simulink model "SimulinkAnalysisofCheetahTail"  (R2022a)
settings: Solver=ode4  StartTime=0.0  StopTime=1.5  FixedStep=0.001  RelTol=1e-3
undefined symbols (not defined in the file): B_cg_H, B_con_H, B_con_L, bar_len, cd_table, Cf, cl_table, g, gear_ratio, int_point_bar, int_point_tail, ITail, M_add, M_cg_H, M_cg_L, M_cg_W, Mb, Mm, Mt, psi3, rho, T_cg_H, T_fur_gap, T_length, T_width_major, T_width_minor, th2_initial, torque_constant, uncertainty_Forces, uncertainty_Position, Vf, windspeed
(part 15 of 21)

== matlab function SimulinkAnalysisofCheetahTail/Model/Forces/NonConstraintForceMatrix_tail_4 ==
  data: B_con_H parameter; B_con_L parameter; Cd input; Cl input; Q_tail_4 output; M_cg_H parameter; M_cg_L parameter; M_cg_W parameter; T_fur_gap parameter; T_length parameter; T_width_major parameter; T_width_minor parameter; area_tail_4_drag input; bar_len parameter; int_point_tail input; psi3 parameter; rho parameter; windspeed parameter; q input; dq input; ddq input
function Q_tail_4 = NonConstraintForceMatrix_tail_4(B_con_H,B_con_L,Cd,Cl,M_cg_H,M_cg_L,M_cg_W,T_fur_gap,T_length,T_width_major,T_width_minor,area_tail_4_drag,bar_len,int_point_tail,psi3,rho,windspeed,q,dq,ddq)
%#codegen
[x,y,z,phi1,th1,psi1,phi2,th2] = deal(q(1),q(2),q(3),q(4),q(5),q(6),q(7),q(8));
[dx,dy,dz,dphi1,dth1,dpsi1,dphi2,dth2] = deal(dq(1),dq(2),dq(3),dq(4),dq(5),dq(6),dq(7),dq(8));
[ddx,ddy,ddz,ddphi1,ddth1,ddpsi1,ddphi2,ddth2] = deal(ddq(1),ddq(2),ddq(3),ddq(4),ddq(5),ddq(6),ddq(7),ddq(8));
%    This function was generated by the Symbolic Math Toolbox version 9.0.
%    17-Feb-2022 12:01:22

t2 = cos(phi1);
t3 = cos(phi2);
t4 = cos(psi1);
t5 = cos(psi3);
t6 = cos(th1);
t7 = cos(th2);
t8 = sin(phi1);
t9 = sin(phi2);
t10 = sin(psi1);
t11 = sin(psi3);
t12 = sin(th1);
t13 = sin(th2);
t14 = M_cg_L+x;
t15 = M_cg_W+y;
t16 = M_cg_H+z;
t19 = -int_point_tail;
t36 = T_length.*(7.0./1.0e+1);
t37 = bar_len.*(7.0./1.0e+1);
t38 = int_point_tail.*(7.0./1.0e+1);
t17 = B_con_L.*t6;
t18 = B_con_L.*t12;
t20 = t2.*t4;
t21 = t6.*t7;
t22 = t2.*t10;
t23 = t4.*t8;
t24 = t7.*t12;
t25 = t8.*t10;
t26 = t12.*t13;
t27 = B_con_H.*t2.*t6;
t29 = t6.*t14;
t30 = B_con_H.*t2.*t12;
t31 = B_con_H.*t6.*t8;
t34 = t12.*t14;
t41 = t6.*t9.*t13;
t43 = t6.*t10.*t13;
t45 = t8.*t9.*t12;
t48 = -t38;
t49 = t2.*t3.*t6;
t50 = T_length+bar_len+t19;
t53 = t2.*t6.*t9;
t54 = t3.*t6.*t8;
t56 = t2.*t6.*t13;
t57 = t3.*t6.*t13;
t59 = t4.*t6.*t13;
t62 = t3.*t8.*t12;
t63 = t6.*t8.*t9;
t68 = t2.*t6.*t15;
t70 = t2.*t6.*t16;
t73 = t6.*t8.*t15;
t74 = t2.*t12.*t16;
t75 = t6.*t8.*t16;
t77 = t8.*t12.*t15;
t105 = t5.*t6.*t8.*t13;
t111 = t6.*t8.*t11.*t13;
t28 = t4.*t17;
t32 = t4.*t18;
t33 = t10.*t17;
t35 = t10.*t18;
t39 = t2.*t26;
t40 = t3.*t26;
t42 = t9.*t24;
t44 = t10.*t24;
t46 = t12.*t25;
t47 = t9.*t26;
t51 = t2.*t21;
t52 = t4.*t21;
t55 = t12.*t20;
t58 = t3.*t24;
t60 = t4.*t24;
t61 = t10.*t21;
t64 = t12.*t22;
t65 = t12.*t23;
t66 = B_con_H.*t6.*t20;
t67 = t4.*t29;
t69 = B_con_H.*t6.*t22;
t71 = t4.*t34;
t72 = t10.*t29;
t76 = t10.*t34;
t78 = -t30;
t79 = -t31;
t81 = -t45;
t86 = t3.*t6.*t23;
t87 = t13.*t49;
t90 = t3.*t8.*t21;
t91 = t6.*t13.*t20;
t92 = t4.*t57;
t95 = t3.*t6.*t25;
t96 = t6.*t9.*t23;
t97 = t2.*t41;
t99 = t8.*t9.*t21;
t100 = t6.*t13.*t22;
t102 = t3.*t43;
t103 = t4.*t41;
t106 = t6.*t9.*t25;
t110 = t10.*t41;
t113 = -t59;
t116 = t6.*t16.*t20;
t117 = t6.*t15.*t23;
t118 = t6.*t16.*t22;
t119 = t6.*t15.*t25;
t120 = -t68;
t121 = -t73;
t122 = -t74;
t123 = -t75;
t124 = t3.*t20.*t21;
t125 = t3.*t21.*t22;
t126 = t9.*t20.*t21;
t127 = t9.*t21.*t22;
t133 = -t105;
t138 = t24+t56;
t212 = t36+t37+t48;
t80 = -t39;
t82 = -t46;
t83 = -t47;
t84 = t3.*t51;
t85 = t3.*t52;
t88 = t2.*t58;
t89 = t9.*t51;
t93 = t3.*t61;
t94 = t9.*t52;
t98 = t2.*t42;
t101 = t4.*t40;
t104 = t9.*t61;
t107 = -t51;
t108 = t10.*t40;
t109 = t4.*t47;
t112 = -t55;
t114 = -t61;
t115 = t10.*t47;
t129 = -t92;
t131 = -t99;
t136 = -t117;
t137 = -t119;
t139 = t22+t65;
t140 = t23+t64;
t141 = -t124;
t142 = -t125;
t149 = t5.*t138;
t153 = t11.*t138;
t157 = t53+t90;
t161 = t58+t87;
t162 = t60+t91;
t163 = t42+t97;
t164 = t44+t100;
t128 = -t84;
t130 = -t93;
t132 = -t104;
t134 = t4.*t83;
t135 = t10.*t83;
t143 = B_con_H.*t139;
t144 = B_con_H.*t140;
t145 = t21+t80;
t146 = t26+t107;
t147 = t20+t82;
t148 = t25+t112;
t150 = t3.*t139;
t151 = t3.*t140;
t152 = t7.*t140;
t154 = t9.*t139;
t155 = t9.*t140;
t156 = t13.*t140;
t165 = t15.*t139;
t166 = t15.*t140;
t167 = t16.*t139;
t168 = t16.*t140;
t174 = t5.*t13.*t139;
t176 = t11.*t13.*t139;
t184 = -t153;
t188 = t49+t131;
t189 = T_fur_gap.*t157;
t190 = T_fur_gap.*t161;
t191 = int_point_tail.*t157;
t192 = int_point_tail.*t161;
t199 = t5.*t162;
t200 = t11.*t162;
t201 = t5.*t163;
t202 = t5.*t164;
t203 = t11.*t163;
t204 = t11.*t164;
t228 = t41+t62+t98;
t231 = t57+t81+t88;
t232 = t54+t83+t89;
t266 = t96+t101+t141;
t268 = t106+t108+t142;
t288 = t157.*t212;
t289 = t161.*t212;
t158 = B_con_H.*t147;
t159 = B_con_H.*t148;
t160 = -t144;
t169 = t7.*t150;
t170 = t7.*t151;
t171 = t13.*t151;
t172 = t7.*t154;
t173 = t9.*t152;
t175 = t13.*t155;
t177 = t5.*t145;
t178 = t5.*t146;
t179 = t3.*t147;
t180 = t3.*t148;
t181 = t7.*t148;
t182 = t11.*t145;
t183 = t11.*t146;
t185 = t9.*t147;
t186 = t9.*t148;
t187 = t13.*t148;
t193 = t15.*t147;
t194 = t15.*t148;
t195 = -t166;
t196 = t16.*t147;
t197 = t16.*t148;
t198 = -t168;
t211 = t5.*t13.*t147;
t214 = t11.*t13.*t147;
t215 = -t176;
t221 = t5.*t188;
t222 = t11.*t188;
t223 = -t204;
t227 = t43+t152;
t229 = t114+t156;
t230 = t40+t63+t128;
t236 = t5.*t228;
t237 = t11.*t228;
t239 = T_fur_gap.*t231;
t240 = T_fur_gap.*t232;
t242 = int_point_tail.*t231;
t243 = int_point_tail.*t232;
t246 = -t5.*(t61-t156);
t249 = -t11.*(t61-t156);
t250 = t5.*t232;
t252 = t11.*t232;
t267 = t86+t126+t134;
t269 = t95+t127+t135;
t276 = T_fur_gap.*t266;
t277 = int_point_tail.*t266;
t278 = T_fur_gap.*t268;
t279 = int_point_tail.*t268;
t306 = t212.*t231;
t307 = t212.*t232;
t340 = t212.*t266;
t343 = t212.*t268;
t370 = t190+t192+t289;
t397 = t79+t120+t123+t189+t191+t288;
t205 = t7.*t179;
t206 = t7.*t180;
t207 = -t169;
t208 = t13.*t180;
t209 = t7.*t185;
t210 = t9.*t181;
t213 = t13.*t186;
t216 = -t177;
t217 = -t179;
t218 = -t183;
t219 = -t193;
t220 = -t194;
t226 = -t214;
t233 = t52+t187;
t234 = t5.*t227;
t235 = t11.*t227;
t238 = T_fur_gap.*t230;
t241 = int_point_tail.*t230;
t244 = t113+t181;
t251 = t12.*t230;
t254 = t130+t171;
t256 = t132+t175;
t257 = t2.*t6.*t230;
t258 = -t5.*(t59-t181);
t259 = t6.*t8.*t230;
t260 = -t11.*(t59-t181);
t262 = -T_fur_gap.*(t93-t171);
t264 = -int_point_tail.*(t93-t171);
t265 = t111+t221;
t270 = -t5.*(t104-t175);
t272 = -t11.*(t104-t175);
t274 = t5.*(t59-t181);
t280 = t133+t222;
t281 = t5.*t269;
t282 = t11.*t269;
t283 = t5.*t267;
t284 = t11.*t267;
t286 = t172+t180;
t290 = t178+t203;
t298 = -T_fur_gap.*(t169-t186);
t300 = -int_point_tail.*(t169-t186);
t302 = t149+t252;
t303 = t102+t170+t185;
t304 = t182+t236;
t305 = t212.*t230;
t311 = t184+t250;
t330 = -t212.*(t93-t171);
t331 = -t12.*(t153-t250);
t337 = -t2.*t6.*(t153-t250);
t338 = -t6.*t8.*(t153-t250);
t346 = t2.*t6.*(t153-t250);
t354 = -t212.*(t169-t186);
t395 = t240+t243+t307;
t396 = t230.*t370;
t401 = -t370.*(t153-t250);
t402 = t370.*(t153-t250);
t404 = -t230.*(t31+t68+t75-t189-t191-t288);
t410 = t17+t29+t77+t78+t122+t239+t242+t306;
t416 = (t153-t250).*(t31+t68+t75-t189-t191-t288);
t432 = t35+t69+t76+t118+t137+t278+t279+t343;
t433 = t32+t66+t71+t116+t136+t276+t277+t340;
t224 = -t205;
t225 = -t210;
t245 = t5.*t233;
t247 = t11.*t233;
t248 = -t234;
t253 = t85+t208;
t255 = t94+t213;
t273 = -t257;
t285 = t151+t209;
t287 = -t283;
t292 = t186+t207;
t294 = t5.*t286;
t296 = t11.*t286;
t301 = t201+t218;
t308 = T_fur_gap.*t303;
t309 = int_point_tail.*t303;
t310 = t129+t154+t206;
t313 = t216+t237;
t314 = t110+t173+t217;
t315 = t12.*t302;
t317 = t5.*t303.*windspeed;
t323 = t2.*t6.*t302;
t324 = t6.*t8.*t302;
t325 = t6.*t10.*t303;
t347 = t199+t284;
t348 = t202+t282;
t350 = t223+t281;
t352 = t140.*t303;
t355 = t235+t270;
t359 = t147.*t303;
t364 = t212.*t303;
t399 = t262+t264+t330;
t400 = t302.*t370;
t403 = t230.*t395;
t409 = t18+t27+t34+t70+t121+t238+t241+t305;
t413 = t302.*t395;
t414 = -t302.*(t31+t68+t75-t189-t191-t288);
t415 = -t395.*(t153-t250);
t417 = t395.*(t153-t250);
t421 = -t416;
t427 = -t303.*(T_fur_gap.*(t93-t171)+int_point_tail.*(t93-t171)+t212.*(t93-t171));
t431 = t303.*(T_fur_gap.*(t93-t171)+int_point_tail.*(t93-t171)+t212.*(t93-t171));
t439 = t230.*t410;
t452 = t302.*t410;
t453 = -t410.*(t153-t250);
t455 = t410.*(t153-t250);
t456 = t143+t167+t220+t298+t300+t354;
t462 = t303.*t432;
t261 = T_fur_gap.*t253;
t263 = int_point_tail.*t253;
t271 = t11.*t255;
t275 = t5.*t255;
t291 = t155+t224;
t293 = t5.*t285;
t295 = t11.*t285;
t312 = t103+t150+t225;
t316 = T_fur_gap.*t310;
t319 = int_point_tail.*t310;
t320 = T_fur_gap.*t314;
t322 = int_point_tail.*t314;
t327 = t212.*t253;
t328 = t5.*t314;
t332 = t11.*t314;
t334 = t11.*t310.*windspeed;
t335 = t19.*t310;
t336 = t4.*t6.*t310;
t339 = -t324;
t349 = t200+t287;
t351 = t174+t296;
t356 = t215+t294;
t358 = t139.*t310;
t360 = t248+t272;
t362 = t148.*t310;
t366 = t212.*t310;
t368 = t212.*t314;
t405 = -t403;
t419 = t157.*t409;
t420 = t161.*t409;
t428 = t231.*t409;
t429 = t232.*t409;
t434 = t5.*t230.*t409;
t435 = t11.*t230.*t409;
t441 = -t439;
t444 = t265.*t409;
t445 = -t409.*(t105-t222);
t447 = t290.*t409;
t448 = -t409.*(t183-t201);
t450 = t304.*t409;
t451 = -t409.*(t177-t237);
t454 = -t452;
t463 = t310.*t433;
t476 = t33+t72+t160+t198+t219+t308+t309+t364;
t478 = -t310.*(-t143-t167+t194+T_fur_gap.*(t169-t186)+int_point_tail.*(t169-t186)+t212.*(t169-t186));
t481 = t310.*(-t143-t167+t194+T_fur_gap.*(t169-t186)+int_point_tail.*(t169-t186)+t212.*(t169-t186));
t297 = T_fur_gap.*t291;
t299 = int_point_tail.*t291;
t318 = T_fur_gap.*t312;
t321 = int_point_tail.*t312;
t326 = t5.*t312;
t329 = t11.*t312;
t333 = -t316;
t341 = -t328;
t344 = -t334;
t345 = -t336;
t353 = t212.*t291;
t357 = t211+t295;
t361 = t226+t293;
t363 = t260+t275;
t365 = t271+t274;
t367 = t212.*t312;
t369 = -t366;
t372 = t246+t332;
t375 = t5.*windspeed.*(t332-t5.*(t61-t156));
t378 = t6.*t10.*(t332-t5.*(t61-t156));
t379 = -t5.*windspeed.*(t328+t11.*(t61-t156));
t384 = -t6.*t10.*(t328+t11.*(t61-t156));
t388 = t140.*(t332-t5.*(t61-t156));
t391 = t147.*(t332-t5.*(t61-t156));
t392 = -t140.*(t328+t11.*(t61-t156));
t394 = -t147.*(t328+t11.*(t61-t156));
t398 = t261+t263+t327;
t418 = t259+t358+t359;
t424 = t273+t352+t362;
t436 = -t428;
t437 = -t429;
t440 = -t435;
t443 = t320+t322+t368;
t446 = -t444;
t449 = -t447;
t459 = -(t332-t5.*(t61-t156)).*(T_fur_gap.*(t93-t171)+int_point_tail.*(t93-t171)+t212.*(t93-t171));
t461 = (t328+t11.*(t61-t156)).*(T_fur_gap.*(t93-t171)+int_point_tail.*(t93-t171)+t212.*(t93-t171));
t465 = -t463;
t483 = t432.*(t332-t5.*(t61-t156));
t493 = -t432.*(t328+t11.*(t61-t156));
t506 = -t476.*(t93-t171);
t507 = t476.*(t93-t171);
t508 = t268.*t476;
t510 = t291.*t476;
t518 = t5.*t303.*t476;
t519 = t11.*t303.*t476;
t520 = t314.*t476;
t522 = t348.*t476;
t524 = -t476.*(t204-t281);
t528 = t355.*t476;
t530 = -t476.*(t234+t11.*(t104-t175));
t532 = -t476.*(t214-t293);
t342 = -t329;
t371 = t247+t326;
t374 = t249+t341;
t385 = -t378;
t406 = t251+t325+t345;
t422 = ddy.*t418;
t423 = dy.*t418;
t425 = ddz.*t424;
t426 = dz.*t424;
t430 = t310.*t398;
t442 = t318+t321+t367;
t458 = t158+t195+t196+t297+t299+t353;
t464 = t303.*t443;
t477 = t28+t67+t159+t165+t197+t333+t335+t369;
t494 = -t483;
t498 = t443.*(t332-t5.*(t61-t156));
t502 = -t443.*(t328+t11.*(t61-t156));
t512 = -t510;
t521 = -t519;
t529 = t357.*t476;
t531 = -t528;
t373 = t245+t342;
t376 = t11.*t371.*windspeed;
t377 = t4.*t6.*t371;
t387 = t139.*t371;
t389 = t148.*t371;
t407 = ddx.*t406;
t408 = dx.*t406;
t438 = -t430;
t457 = t371.*t398;
t466 = t310.*t442;
t479 = t303.*t458;
t484 = t371.*t433;
t499 = t371.*t442;
t509 = t253.*t477;
t511 = t266.*t477;
t513 = -t371.*(-t143-t167+t194+T_fur_gap.*(t169-t186)+int_point_tail.*(t169-t186)+t212.*(t169-t186));
t515 = t458.*(t332-t5.*(t61-t156));
t516 = -t458.*(t328+t11.*(t61-t156));
t517 = -t477.*(t169-t186);
t523 = t312.*t477;
t525 = t5.*t310.*t477;
t526 = t11.*t310.*t477;
t533 = -t529;
t534 = t347.*t477;
t535 = t349.*t477;
t536 = t351.*t477;
t538 = -t477.*(t176-t294);
t539 = t477.*(t176-t294);
t540 = t363.*t477;
t541 = t365.*t477;
Q_tail_4 = ft_1({Cd,Cl,T_fur_gap,T_width_major,T_width_minor,area_tail_4_drag,ddphi1,ddphi2,ddth1,ddth2,ddx,ddy,ddz,dphi1,dphi2,dth1,dth2,dx,dy,dz,int_point_tail,rho,t10,t104,t105,t11,t12,t138,t139,t140,t143,t147,t148,t153,t156,t167,t169,t171,t175,t177,t186,t189,t191,t194,t2,t204,t212,t214,t222,t230,t232,t233,t234,t237,t250,t281,t288,t293,t302,t303,t31,t310,t312,t314,t315,t317,t323,t328,t331,t332,t338,t339,t344,t346,t370,t371,t373,t375,t376,t377,t379,t384,t385,t387,t388,t389,t391,t392,t394,t395,t396,t398,t4,t400,t402,t403,t404,t405,t407,t408,t409,t410,t413,t414,t415,t416,t417,t419,t420,t421,t422,t423,t425,t426,t428,t429,t431,t432,t433,t434,t436,t437,t438,t439,t440,t441,t442,t443,t444,t445,t446,t447,t448,t449,t450,t451,t452,t453,t454,t455,t457,t458,t459,t461,t462,t463,t464,t465,t466,t476,t477,t478,t479,t481,t483,t484,t493,t494,t498,t499,t5,t50,t502,t507,t508,t509,t510,t511,t512,t513,t515,t516,t517,t518,t520,t521,t522,t523,t524,t525,t526,t529,t530,t531,t532,t533,t534,t535,t536,t538,t539,t540,t541,t6,t61,t68,t75,t8,t93,th2,windspeed});
end
function Q_tail_4 = ft_1(ct)
Cd = ct{1};
Cl = ct{2};
T_fur_gap = ct{3};
T_width_major = ct{4};
T_width_minor = ct{5};
area_tail_4_drag = ct{6};
ddphi1 = ct{7};
ddphi2 = ct{8};
ddth1 = ct{9};
ddth2 = ct{10};
ddx = ct{11};
ddy = ct{12};
ddz = ct{13};
dphi1 = ct{14};
dphi2 = ct{15};
dth1 = ct{16};
dth2 = ct{17};
dx = ct{18};
dy = ct{19};
dz = ct{20};
int_point_tail = ct{21};
rho = ct{22};
t10 = ct{23};
t104 = ct{24};
t105 = ct{25};
t11 = ct{26};
t12 = ct{27};
t138 = ct{28};
t139 = ct{29};
t140 = ct{30};
t143 = ct{31};
t147 = ct{32};
t148 = ct{33};
t153 = ct{34};
t156 = ct{35};
t167 = ct{36};
t169 = ct{37};
t171 = ct{38};
t175 = ct{39};
t177 = ct{40};
t186 = ct{41};
t189 = ct{42};
t191 = ct{43};
t194 = ct{44};
t2 = ct{45};
t204 = ct{46};
t212 = ct{47};
t214 = ct{48};
t222 = ct{49};
t230 = ct{50};
t232 = ct{51};
t233 = ct{52};
t234 = ct{53};
t237 = ct{54};
t250 = ct{55};
t281 = ct{56};
t288 = ct{57};
t293 = ct{58};
t302 = ct{59};
t303 = ct{60};
t31 = ct{61};
t310 = ct{62};
t312 = ct{63};
t314 = ct{64};
t315 = ct{65};
t317 = ct{66};
t323 = ct{67};
t328 = ct{68};
t331 = ct{69};
t332 = ct{70};
t338 = ct{71};
t339 = ct{72};
t344 = ct{73};
t346 = ct{74};
t370 = ct{75};
t371 = ct{76};
t373 = ct{77};
t375 = ct{78};
t376 = ct{79};
t377 = ct{80};
t379 = ct{81};
t384 = ct{82};
t385 = ct{83};
t387 = ct{84};
t388 = ct{85};
t389 = ct{86};
t391 = ct{87};
t392 = ct{88};
t394 = ct{89};
t395 = ct{90};
t396 = ct{91};
t398 = ct{92};
t4 = ct{93};
t400 = ct{94};
t402 = ct{95};
t403 = ct{96};
t404 = ct{97};
t405 = ct{98};
t407 = ct{99};
t408 = ct{100};
t409 = ct{101};
t410 = ct{102};
t413 = ct{103};
t414 = ct{104};
t415 = ct{105};
t416 = ct{106};
t417 = ct{107};
t419 = ct{108};
t420 = ct{109};
t421 = ct{110};
t422 = ct{111};
t423 = ct{112};
t425 = ct{113};
t426 = ct{114};
t428 = ct{115};
t429 = ct{116};
t431 = ct{117};
t432 = ct{118};
t433 = ct{119};
t434 = ct{120};
t436 = ct{121};
t437 = ct{122};
t438 = ct{123};
t439 = ct{124};
t440 = ct{125};
t441 = ct{126};
t442 = ct{127};
t443 = ct{128};
t444 = ct{129};
t445 = ct{130};
t446 = ct{131};
t447 = ct{132};
t448 = ct{133};
t449 = ct{134};
t450 = ct{135};
t451 = ct{136};
t452 = ct{137};
t453 = ct{138};
t454 = ct{139};
t455 = ct{140};
t457 = ct{141};
t458 = ct{142};
t459 = ct{143};
t461 = ct{144};
t462 = ct{145};
t463 = ct{146};
t464 = ct{147};
t465 = ct{148};
t466 = ct{149};
t476 = ct{150};
t477 = ct{151};
t478 = ct{152};
t479 = ct{153};
t481 = ct{154};
t483 = ct{155};
t484 = ct{156};
t493 = ct{157};
t494 = ct{158};
t498 = ct{159};
t499 = ct{160};
t5 = ct{161};
t50 = ct{162};
t502 = ct{163};
t507 = ct{164};
t508 = ct{165};
t509 = ct{166};
t510 = ct{167};
t511 = ct{168};
t512 = ct{169};
t513 = ct{170};
t515 = ct{171};
t516 = ct{172};
t517 = ct{173};
t518 = ct{174};
t520 = ct{175};
t521 = ct{176};
t522 = ct{177};
t523 = ct{178};
t524 = ct{179};
t525 = ct{180};
t526 = ct{181};
t529 = ct{182};
t530 = ct{183};
t531 = ct{184};
t532 = ct{185};
t533 = ct{186};
t534 = ct{187};
t535 = ct{188};
t536 = ct{189};
t538 = ct{190};
t539 = ct{191};
t540 = ct{192};
t541 = ct{193};
t6 = ct{194};
t61 = ct{195};
t68 = ct{196};
t75 = ct{197};
t8 = ct{198};
t93 = ct{199};
th2 = ct{200};
windspeed = ct{201};
t380 = t11.*t373.*windspeed;
t381 = -t376;
t382 = t4.*t6.*t373;
t383 = -t377;
t390 = t139.*t373;
t393 = t148.*t373;
t411 = -t407;
t412 = -t408;
t460 = t373.*t398;
t467 = -t466;
t472 = -ddx.*(t377+t12.*(t153-t250)+t6.*t10.*(t328+t11.*(t61-t156)));
t473 = -dx.*(t377+t12.*(t153-t250)+t6.*t10.*(t328+t11.*(t61-t156)));
t474 = ddx.*(t377+t12.*(t153-t250)+t6.*t10.*(t328+t11.*(t61-t156)));
t475 = dx.*(t377+t12.*(t153-t250)+t6.*t10.*(t328+t11.*(t61-t156)));
t482 = -t479;
t485 = t338+t387+t394;
t489 = -ddy.*(-t387+t147.*(t328+t11.*(t61-t156))+t6.*t8.*(t153-t250));
t491 = -dy.*(-t387+t147.*(t328+t11.*(t61-t156))+t6.*t8.*(t153-t250));
t495 = t373.*t433;
t496 = -t484;
t497 = t346+t389+t392;
t503 = t373.*t442;
t504 = -t499;
t514 = -t373.*(-t143-t167+t194+T_fur_gap.*(t169-t186)+int_point_tail.*(t169-t186)+t212.*(t169-t186));
t527 = -t525;
t537 = -t535;
t542 = -t541;
t543 = t396+t420+t431+t438+t507+t509;
t548 = t436+t441+t462+t465+t508+t511;
t549 = -ddth1.*(t428+t439-t462+t463-t508-t511);
t550 = -dth1.*(t428+t439-t462+t463-t508-t511);
t552 = t402+t448+t457+t461+t531+t540;
t554 = -ddphi2.*(t403+t429-t464+t466-t520-t523);
t555 = -dphi2.*(t403+t429-t464+t466-t520-t523);
t561 = -ddphi1.*(-t419+t478+t479+t510+t230.*(t31+t68+t75-t189-t191-t288)+t477.*(t169-t186));
t562 = -dphi1.*(-t419+t478+t479+t510+t230.*(t31+t68+t75-t189-t191-t288)+t477.*(t169-t186));
t563 = ddphi1.*(-t419+t478+t479+t510+t230.*(t31+t68+t75-t189-t191-t288)+t477.*(t169-t186));
t564 = dphi1.*(-t419+t478+t479+t510+t230.*(t31+t68+t75-t189-t191-t288)+t477.*(t169-t186));
t569 = -ddphi2.*(t415-t434+t499-t518+t525+t443.*(t328+t11.*(t61-t156)));
t570 = -dphi2.*(t415-t434+t499-t518+t525+t443.*(t328+t11.*(t61-t156)));
t577 = -ddth1.*(-t450+t453+t484+t535+t432.*(t328+t11.*(t61-t156))+t476.*(t204-t281));
t578 = -dth1.*(-t450+t453+t484+t535+t432.*(t328+t11.*(t61-t156))+t476.*(t204-t281));
t580 = -ddphi1.*(-t515+t529-t536+t302.*(t31+t68+t75-t189-t191-t288)+t409.*(t105-t222)+t373.*(-t143-t167+t194+T_fur_gap.*(t169-t186)+int_point_tail.*(t169-t186)+t212.*(t169-t186)));
t581 = -dphi1.*(-t515+t529-t536+t302.*(t31+t68+t75-t189-t191-t288)+t409.*(t105-t222)+t373.*(-t143-t167+t194+T_fur_gap.*(t169-t186)+int_point_tail.*(t169-t186)+t212.*(t169-t186)));
t582 = t421+t446+t513+t516+t532+t539;
t583 = -ddphi1.*(t416+t444+t538+t458.*(t328+t11.*(t61-t156))+t476.*(t214-t293)+t371.*(-t143-t167+t194+T_fur_gap.*(t169-t186)+int_point_tail.*(t169-t186)+t212.*(t169-t186)));
t584 = -dphi1.*(t416+t444+t538+t458.*(t328+t11.*(t61-t156))+t476.*(t214-t293)+t371.*(-t143-t167+t194+T_fur_gap.*(t169-t186)+int_point_tail.*(t169-t186)+t212.*(t169-t186)));
t386 = -t380;
t468 = t315+t382+t385;
t471 = t331+t383+t384;
t480 = t323+t388+t393;
t486 = t339+t390+t391;
t500 = ddz.*t497;
t501 = dz.*t497;
t505 = -t503;
t544 = ddth2.*t543;
t545 = dth2.*t543;
t551 = t405+t437+t464+t467+t520+t523;
t553 = t400+t449+t459+t460+t530+t542;
t556 = ddth2.*t552;
t557 = -ddth2.*(-t400+t447-t460+t541+t476.*(t234+t11.*(t104-t175))+(t332-t5.*(t61-t156)).*(T_fur_gap.*(t93-t171)+int_point_tail.*(t93-t171)+t212.*(t93-t171)));
t558 = dth2.*t552;
t559 = -dth2.*(-t400+t447-t460+t541+t476.*(t234+t11.*(t104-t175))+(t332-t5.*(t61-t156)).*(T_fur_gap.*(t93-t171)+int_point_tail.*(t93-t171)+t212.*(t93-t171)));
t560 = t404+t419+t481+t482+t512+t517;
t568 = t417+t434+t502+t504+t518+t527;
t571 = t451+t454+t494+t495+t522+t534;
t572 = -ddth1.*(t452+t483-t495-t522-t534+t409.*(t177-t237));
t573 = -dth1.*(t452+t483-t495-t522-t534+t409.*(t177-t237));
t574 = ddth1.*(t452+t483-t495-t522-t534+t409.*(t177-t237));
t575 = dth1.*(t452+t483-t495-t522-t534+t409.*(t177-t237));
t576 = t450+t455+t493+t496+t524+t537;
t579 = t414+t445+t514+t515+t533+t536;
t469 = ddx.*t468;
t470 = dx.*t468;
t487 = ddz.*t480;
t488 = dz.*t480;
t490 = ddy.*t486;
t492 = dy.*t486;
t546 = -t544;
t547 = -t545;
t565 = t413+t440+t498+t505+t521+t526;
t594 = t474+t489+t500+t556+t569+t577+t583;
t600 = t379+t381+t475+t491+t501+t558+t570+t578+t584;
t602 = -1.0./(t376+t473-t501-t558+dy.*(-t387+t147.*(t328+t11.*(t61-t156))+t6.*t8.*(t153-t250))+dphi2.*(t415-t434+t499-t518+t525+t443.*(t328+t11.*(t61-t156)))+dphi1.*(t416+t444+t538+t458.*(t328+t11.*(t61-t156))+t476.*(t214-t293)+t371.*(-t143-t167+t194+T_fur_gap.*(t169-t186)+int_point_tail.*(t169-t186)+t212.*(t169-t186)))+dth1.*(-t450+t453+t484+t535+t432.*(t328+t11.*(t61-t156))+t476.*(t204-t281))+t5.*windspeed.*(t328+t11.*(t61-t156)));
t566 = ddphi2.*t565;
t567 = dphi2.*t565;
t585 = t411+t422+t425+t546+t549+t554+t563;
t588 = t317+t344+t412+t423+t426+t547+t550+t555+t564;
t595 = abs(t594);
t601 = abs(t600);
t586 = abs(t585);
t589 = abs(t588);
t591 = t469+t487+t490+t557+t566+t574+t580;
t596 = t595.^2;
t597 = t375+t386+t470+t488+t492+t559+t567+t575+t581;
t603 = t601.^2;
t604 = t588.*t602;
t587 = t586.^2;
t590 = t589.^2;
t592 = abs(t591);
t598 = abs(t597);
t605 = atan(t604);
t593 = t592.^2;
t599 = t598.^2;
t606 = -t605;
t607 = t606+th2;
t609 = t587+t593+t596;
t612 = t590+t599+t603;
t608 = cos(t607);
t610 = sqrt(t609);
t613 = sqrt(t612);
t611 = (T_width_major.*T_width_minor.*rho.*t50.*t610.*pi)./2.0e+1;
t614 = 1.0./t613;
t615 = (Cd.*area_tail_4_drag.*rho.*t608.*t612)./2.0;
t616 = (Cl.*T_width_major.*T_width_minor.*rho.*t588.*t608.*t613.*pi)./2.0;
t617 = Cl.*T_width_major.*T_width_minor.*rho.*t588.*t608.*t613.*pi.*3.061616997868383e-17;
t618 = (Cl.*T_width_major.*T_width_minor.*rho.*t138.*t597.*t608.*t613.*pi)./2.0;
t619 = Cl.*T_width_major.*T_width_minor.*rho.*t608.*t613.*pi.*(t376+t473-t501-t558+dy.*(-t387+t147.*(t328+t11.*(t61-t156))+t6.*t8.*(t153-t250))+dphi2.*(t415-t434+t499-t518+t525+t443.*(t328+t11.*(t61-t156)))+dphi1.*(t416+t444+t538+t458.*(t328+t11.*(t61-t156))+t476.*(t214-t293)+t371.*(-t143-t167+t194+T_fur_gap.*(t169-t186)+int_point_tail.*(t169-t186)+t212.*(t169-t186)))+dth1.*(-t450+t453+t484+t535+t432.*(t328+t11.*(t61-t156))+t476.*(t204-t281))+t5.*windspeed.*(t328+t11.*(t61-t156))).*(-1.0./2.0);
t620 = (Cl.*T_width_major.*T_width_minor.*rho.*t233.*t597.*t608.*t613.*pi)./2.0;
t621 = Cl.*T_width_major.*T_width_minor.*rho.*t597.*t608.*t613.*pi.*(t61-t156).*(-1.0./2.0);
et1 = Cl.*T_width_major.*T_width_minor.*rho.*t608.*t613.*pi.*(t376+t473-t501-t558+dy.*(-t387+t147.*(t328+t11.*(t61-t156))+t6.*t8.*(t153-t250))+dphi2.*(t415-t434+t499-t518+t525+t443.*(t328+t11.*(t61-t156)))+dphi1.*(t416+t444+t538+t458.*(t328+t11.*(t61-t156))+t476.*(t214-t293)+t371.*(-t143-t167+t194+T_fur_gap.*(t169-t186)+int_point_tail.*(t169-t186)+t212.*(t169-t186)))+dth1.*(-t450+t453+t484+t535+t432.*(t328+t11.*(t61-t156))+t476.*(t204-t281))+t5.*windspeed.*(t328+t11.*(t61-t156)));
et2 = -3.061616997868383e-17;
t622 = et1.*et2;
et3 = Cl.*T_width_major.*T_width_minor.*rho.*t608.*t613.*pi.*(t376+t473-t501-t558+dy.*(-t387+t147.*(t328+t11.*(t61-t156))+t6.*t8.*(t153-t250))+dphi2.*(t415-t434+t499-t518+t525+t443.*(t328+t11.*(t61-t156)))+dphi1.*(t416+t444+t538+t458.*(t328+t11.*(t61-t156))+t476.*(t214-t293)+t371.*(-t143-t167+t194+T_fur_gap.*(t169-t186)+int_point_tail.*(t169-t186)+t212.*(t169-t186)))+dth1.*(-t450+t453+t484+t535+t432.*(t328+t11.*(t61-t156))+t476.*(t204-t281))+t5.*windspeed.*(t328+t11.*(t61-t156)));
et4 = 3.061616997868383e-17;
t623 = et3.*et4;
t624 = t611+t615;
t628 = t617+t619;
t629 = t616+t623;
t625 = t230.*t588.*t614.*t624;
t626 = t303.*t588.*t614.*t624;
t627 = t310.*t588.*t614.*t624;
t630 = t230.*t628;
t631 = t232.*t629;
t633 = t303.*t628;
t634 = t310.*t628;
t635 = t312.*t629;
t636 = t314.*t629;
t638 = t138.*t597.*t614.*t624;
t640 = t233.*t597.*t614.*t624;
t641 = -t597.*t614.*t624.*(t61-t156);
t642 = -t232.*t614.*t624.*(t376+t473-t501-t558+dy.*(-t387+t147.*(t328+t11.*(t61-t156))+t6.*t8.*(t153-t250))+dphi2.*(t415-t434+t499-t518+t525+t443.*(t328+t11.*(t61-t156)))+dphi1.*(t416+t444+t538+t458.*(t328+t11.*(t61-t156))+t476.*(t214-t293)+t371.*(-t143-t167+t194+T_fur_gap.*(t169-t186)+int_point_tail.*(t169-t186)+t212.*(t169-t186)))+dth1.*(-t450+t453+t484+t535+t432.*(t328+t11.*(t61-t156))+t476.*(t204-t281))+t5.*windspeed.*(t328+t11.*(t61-t156)));
t643 = -t312.*t614.*t624.*(t376+t473-t501-t558+dy.*(-t387+t147.*(t328+t11.*(t61-t156))+t6.*t8.*(t153-t250))+dphi2.*(t415-t434+t499-t518+t525+t443.*(t328+t11.*(t61-t156)))+dphi1.*(t416+t444+t538+t458.*(t328+t11.*(t61-t156))+t476.*(t214-t293)+t371.*(-t143-t167+t194+T_fur_gap.*(t169-t186)+int_point_tail.*(t169-t186)+t212.*(t169-t186)))+dth1.*(-t450+t453+t484+t535+t432.*(t328+t11.*(t61-t156))+t476.*(t204-t281))+t5.*windspeed.*(t328+t11.*(t61-t156)));
t644 = -t314.*t614.*t624.*(t376+t473-t501-t558+dy.*(-t387+t147.*(t328+t11.*(t61-t156))+t6.*t8.*(t153-t250))+dphi2.*(t415-t434+t499-t518+t525+t443.*(t328+t11.*(t61-t156)))+dphi1.*(t416+t444+t538+t458.*(t328+t11.*(t61-t156))+t476.*(t214-t293)+t371.*(-t143-t167+t194+T_fur_gap.*(t169-t186)+int_point_tail.*(t169-t186)+t212.*(t169-t186)))+dth1.*(-t450+t453+t484+t535+t432.*(t328+t11.*(t61-t156))+t476.*(t204-t281))+t5.*windspeed.*(t328+t11.*(t61-t156)));
t645 = t314.*t614.*t624.*(t376+t473-t501-t558+dy.*(-t387+t147.*(t328+t11.*(t61-t156))+t6.*t8.*(t153-t250))+dphi2.*(t415-t434+t499-t518+t525+t443.*(t328+t11.*(t61-t156)))+dphi1.*(t416+t444+t538+t458.*(t328+t11.*(t61-t156))+t476.*(t214-t293)+t371.*(-t143-t167+t194+T_fur_gap.*(t169-t186)+int_point_tail.*(t169-t186)+t212.*(t169-t186)))+dth1.*(-t450+t453+t484+t535+t432.*(t328+t11.*(t61-t156))+t476.*(t204-t281))+t5.*windspeed.*(t328+t11.*(t61-t156)));
t632 = -t630;
t637 = -t635;
t639 = -t638;
t647 = t621+t633+t636;
t650 = t627+t640+t643;
t651 = t626+t641+t645;
t646 = t618+t631+t632;
t648 = t620+t634+t637;
t649 = t625+t639+t642;
et5 = -t12.*t646+t12.*(-t625+t638+t232.*t614.*t624.*(t376+t473-t501-t558+dy.*(-t387+t147.*(t328+t11.*(t61-t156))+t6.*t8.*(t153-t250))+dphi2.*(t415-t434+t499-t518+t525+t443.*(t328+t11.*(t61-t156)))+dphi1.*(t416+t444+t538+t458.*(t328+t11.*(t61-t156))+t476.*(t214-t293)+t371.*(-t143-t167+t194+T_fur_gap.*(t169-t186)+int_point_tail.*(t169-t186)+t212.*(t169-t186)))+dth1.*(-t450+t453+t484+t535+t432.*(t328+t11.*(t61-t156))+t476.*(t204-t281))+t5.*windspeed.*(t328+t11.*(t61-t156))))-t4.*t6.*t648+t4.*t6.*t650;
et6 = t6.*t10.*t647-t6.*t10.*t651;
et7 = -t139.*t648+t139.*t650-t147.*t647+t147.*t651;
et8 = -t6.*t8.*(-t625+t638+t232.*t614.*t624.*(t376+t473-t501-t558+dy.*(-t387+t147.*(t328+t11.*(t61-t156))+t6.*t8.*(t153-t250))+dphi2.*(t415-t434+t499-t518+t525+t443.*(t328+t11.*(t61-t156)))+dphi1.*(t416+t444+t538+t458.*(t328+t11.*(t61-t156))+t476.*(t214-t293)+t371.*(-t143-t167+t194+T_fur_gap.*(t169-t186)+int_point_tail.*(t169-t186)+t212.*(t169-t186)))+dth1.*(-t450+t453+t484+t535+t432.*(t328+t11.*(t61-t156))+t476.*(t204-t281))+t5.*windspeed.*(t328+t11.*(t61-t156))))+t6.*t8.*t646;
et9 = -t140.*t647+t140.*t651-t148.*t648+t148.*t650+t2.*t6.*(-t625+t638+t232.*t614.*t624.*(t376+t473-t501-t558+dy.*(-t387+t147.*(t328+t11.*(t61-t156))+t6.*t8.*(t153-t250))+dphi2.*(t415-t434+t499-t518+t525+t443.*(t328+t11.*(t61-t156)))+dphi1.*(t416+t444+t538+t458.*(t328+t11.*(t61-t156))+t476.*(t214-t293)+t371.*(-t143-t167+t194+T_fur_gap.*(t169-t186)+int_point_tail.*(t169-t186)+t212.*(t169-t186)))+dth1.*(-t450+t453+t484+t535+t432.*(t328+t11.*(t61-t156))+t476.*(t204-t281))+t5.*windspeed.*(t328+t11.*(t61-t156))));
et10 = -t2.*t6.*t646;
et11 = t646.*(t31+t68+t75-t189-t191-t288)-t458.*t647+t458.*t651;
et12 = -(-t625+t638+t232.*t614.*t624.*(t376+t473-t501-t558+dy.*(-t387+t147.*(t328+t11.*(t61-t156))+t6.*t8.*(t153-t250))+dphi2.*(t415-t434+t499-t518+t525+t443.*(t328+t11.*(t61-t156)))+dphi1.*(t416+t444+t538+t458.*(t328+t11.*(t61-t156))+t476.*(t214-t293)+t371.*(-t143-t167+t194+T_fur_gap.*(t169-t186)+int_point_tail.*(t169-t186)+t212.*(t169-t186)))+dth1.*(-t450+t453+t484+t535+t432.*(t328+t11.*(t61-t156))+t476.*(t204-t281))+t5.*windspeed.*(t328+t11.*(t61-t156)))).*(t31+t68+t75-t189-t191-t288);
et13 = t648.*(-t143-t167+t194+T_fur_gap.*(t169-t186)+int_point_tail.*(t169-t186)+t212.*(t169-t186))-t650.*(-t143-t167+t194+T_fur_gap.*(t169-t186)+int_point_tail.*(t169-t186)+t212.*(t169-t186));
et14 = -t410.*t646-t432.*t647+t433.*t648+t432.*t651-t433.*t650;
et15 = t410.*(-t625+t638+t232.*t614.*t624.*(t376+t473-t501-t558+dy.*(-t387+t147.*(t328+t11.*(t61-t156))+t6.*t8.*(t153-t250))+dphi2.*(t415-t434+t499-t518+t525+t443.*(t328+t11.*(t61-t156)))+dphi1.*(t416+t444+t538+t458.*(t328+t11.*(t61-t156))+t476.*(t214-t293)+t371.*(-t143-t167+t194+T_fur_gap.*(t169-t186)+int_point_tail.*(t169-t186)+t212.*(t169-t186)))+dth1.*(-t450+t453+t484+t535+t432.*(t328+t11.*(t61-t156))+t476.*(t204-t281))+t5.*windspeed.*(t328+t11.*(t61-t156))));
et16 = -t395.*t646+t442.*t648-t443.*t647-t442.*t650+t443.*t651;
et17 = t395.*(-t625+t638+t232.*t614.*t624.*(t376+t473-t501-t558+dy.*(-t387+t147.*(t328+t11.*(t61-t156))+t6.*t8.*(t153-t250))+dphi2.*(t415-t434+t499-t518+t525+t443.*(t328+t11.*(t61-t156)))+dphi1.*(t416+t444+t538+t458.*(t328+t11.*(t61-t156))+t476.*(t214-t293)+t371.*(-t143-t167+t194+T_fur_gap.*(t169-t186)+int_point_tail.*(t169-t186)+t212.*(t169-t186)))+dth1.*(-t450+t453+t484+t535+t432.*(t328+t11.*(t61-t156))+t476.*(t204-t281))+t5.*windspeed.*(t328+t11.*(t61-t156))));
et18 = -t370.*t646-t398.*t648+t398.*t650+t647.*(T_fur_gap.*(t93-t171)+int_point_tail.*(t93-t171)+t212.*(t93-t171))-t651.*(T_fur_gap.*(t93-t171)+int_point_tail.*(t93-t171)+t212.*(t93-t171));
et19 = t370.*(-t625+t638+t232.*t614.*t624.*(t376+t473-t501-t558+dy.*(-t387+t147.*(t328+t11.*(t61-t156))+t6.*t8.*(t153-t250))+dphi2.*(t415-t434+t499-t518+t525+t443.*(t328+t11.*(t61-t156)))+dphi1.*(t416+t444+t538+t458.*(t328+t11.*(t61-t156))+t476.*(t214-t293)+t371.*(-t143-t167+t194+T_fur_gap.*(t169-t186)+int_point_tail.*(t169-t186)+t212.*(t169-t186)))+dth1.*(-t450+t453+t484+t535+t432.*(t328+t11.*(t61-t156))+t476.*(t204-t281))+t5.*windspeed.*(t328+t11.*(t61-t156))));
Q_tail_4 = [et5+et6;et7+et8;et9+et10;et11+et12+et13;et14+et15;t476.*t648+t477.*t647-t476.*t650-t477.*t651;et16+et17;et18+et19];
end
